simulink subsystem "Mag"  (R2022a)
settings: Solver=VariableStepAuto  StartTime=0.0  StopTime=10.0  RelTol=1e-3
undefined symbols (not defined in the file or in its folder): sig_mag
libraries: matrix_library x2
settings Model: Creator=emmamarsden  LastModifiedBy=emmamarsden

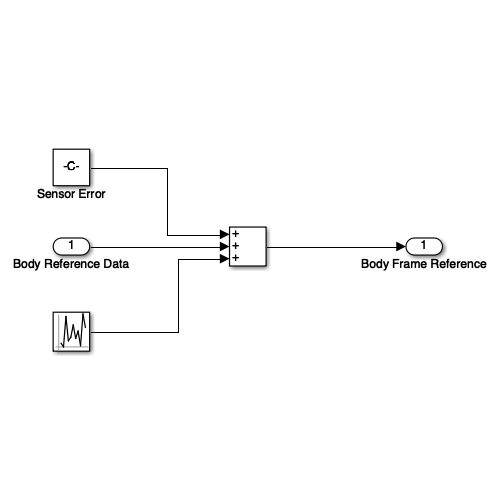
[thumbnail: Simulink's stored preview of the top-level diagram]
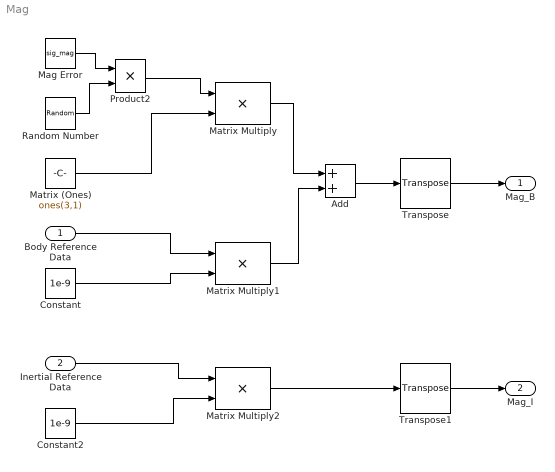
== system Mag ==
  Body Reference Data : Inport
  Inertial Reference Data : Inport  Port=2
  Add : Sum
  Constant : Constant  Value=1e-9
  Constant2 : Constant  Value=1e-9
  Mag Error : Constant  Value=sig_mag
  Matrix (Ones) : Constant  Value=ones(3,1)  VectorParams1D=off
  Matrix Multiply : Product
  Matrix Multiply1 : Product
  Matrix Multiply2 : Product
  Product2 : Product
  "Random Number " : UniformRandomNumber  SampleTime=0.1
  Transpose : matrix_library/Transpose
      settings: SourceProductBaseCode=SL
  Transpose1 : matrix_library/Transpose
      settings: SourceProductBaseCode=SL
  Mag_B : Outport
  Mag_I : Outport  Port=2
  wires:
  Transpose1/1 -> Mag_I/1
  Matrix Multiply1/1 -> Add/2
  Matrix Multiply/1 -> Add/1
  "Random Number "/1 -> Product2/2
  Matrix (Ones)/1 -> Matrix Multiply/2
  Product2/1 -> Matrix Multiply/1
  Mag Error/1 -> Product2/1
  Constant/1 -> Matrix Multiply1/2
  Add/1 -> Transpose/1
  Transpose/1 -> Mag_B/1
  Body Reference Data/1 -> Matrix Multiply1/1
  Constant2/1 -> Matrix Multiply2/2
  Inertial Reference Data/1 -> Matrix Multiply2/1
  Matrix Multiply2/1 -> Transpose1/1
